simulink model "part7_"  (R2021b)
settings: Solver=VariableStepAuto  StartTime=0.0  StopTime=10.0  RelTol=1e-3
settings Model: Creator=aaomi  LastModifiedBy=aaomi

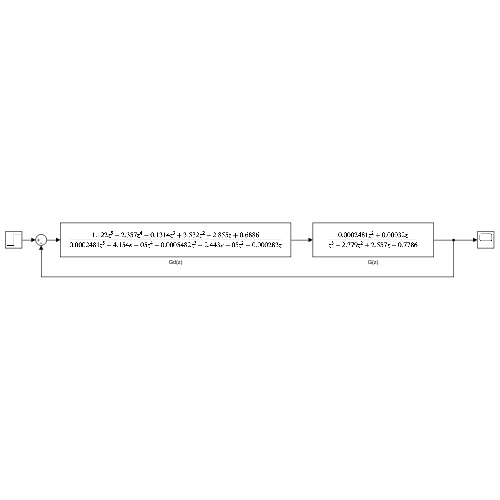
[thumbnail: Simulink's stored preview of the top-level diagram]
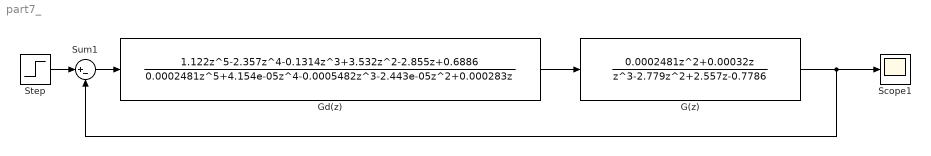
== system part7_ ==
  G(z) : DiscreteTransferFcn  Numerator=[0.0002481 0.00032 0]  Denominator=[1 -2.779 2.557 -0.7786]
  Gd(z) : DiscreteTransferFcn  Numerator=[1.122 -2.357 -0.1314 3.532 -2.855 0.6886]  Denominator=[0.0002481 4.154e-05 -0.0005482 -2.443e-05 0.000283 0]
  Scope1 : Scope
  Step : Step  SampleTime=0
  Sum1 : Sum  Inputs=|+-
  wires:
  G(z)/1 -> Sum1/2, Scope1/1
  Step/1 -> Sum1/1
  Sum1/1 -> Gd(z)/1
  Gd(z)/1 -> G(z)/1
